simulink model "exp_3"  (R2024b)
settings: Solver=FixedStepAuto  StartTime=0.0  StopTime=0.02  FixedStep=0.0001  RelTol=1e-3
settings Model: Creator=乔钰理  LastModifiedBy=86195
settings RTWCC: GPUComputeCapability=3.5

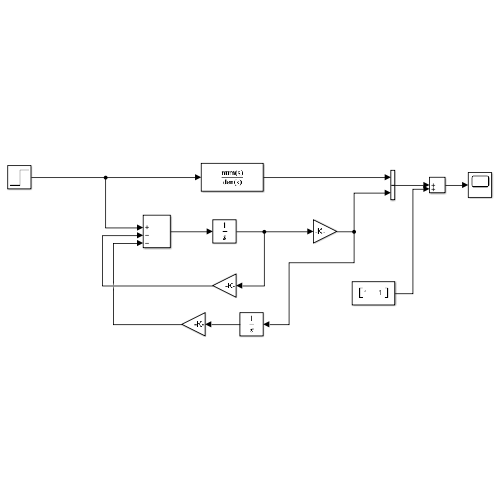
[thumbnail: Simulink's stored preview of the top-level diagram]
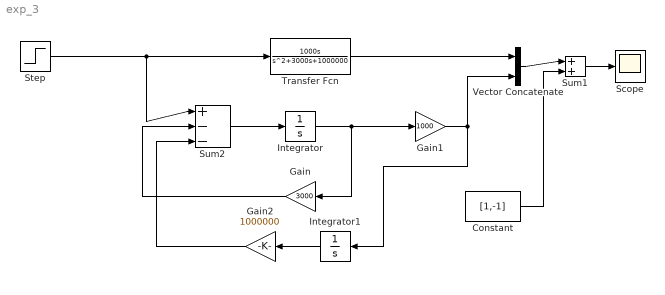
== system exp_3 ==
  Constant : Constant  Value=[1,-1]
  Gain : Gain  Gain=3000
  Gain1 : Gain  Gain=1000
  Gain2 : Gain  Gain=1000000
  Integrator : Integrator
  Integrator1 : Integrator
  Scope : Scope
  Step : Step  SampleTime=0
  Sum1 : Sum  Inputs=|++
  Sum2 : Sum  Inputs=|+--
  Transfer Fcn : TransferFcn  Numerator=[1000 0]  Denominator=[1 3000 1000000]
  Vector Concatenate : Concatenate
  wires:
  Step/1 -> Transfer Fcn/1, Sum2/1
  Sum2/1 -> Integrator/1
  Sum1/1 -> Scope/1
  Constant/1 -> Sum1/2
  Integrator/1 -> Gain/1, Gain1/1
  Gain1/1 -> Integrator1/1, Vector Concatenate/2
  Transfer Fcn/1 -> Vector Concatenate/1
  Vector Concatenate/1 -> Sum1/1
  Gain/1 -> Sum2/2
  Integrator1/1 -> Gain2/1
  Gain2/1 -> Sum2/3
